simulink model "SensorTesting"  (R2025a)
settings: Solver=VariableStepAuto  StartTime=0.0  StopTime=10.0  RelTol=1e-3
undefined symbols (not defined in the file): fractalcoef
libraries: sensorgpslib x1, mspsensorlib x1, simulink x1
settings Model: Creator=jonno  LastModifiedBy=jonno

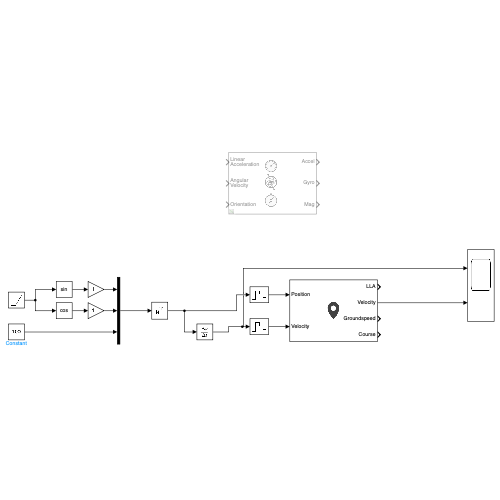
[thumbnail: Simulink's stored preview of the top-level diagram]
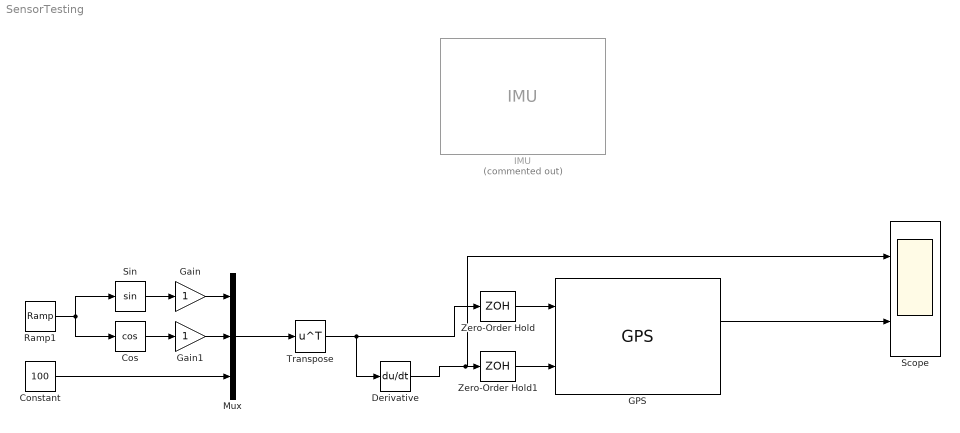
== system SensorTesting ==
  Constant : Constant  Value=100
  Cos : Trigonometry  Operator=cos
  Derivative : Derivative
  GPS : sensorgpslib/GPS  DispRefFrame=NED  PositionInputFormat=Local  ReferenceLocation=[ 0, 0, 0 ]  HorizontalPositionAccuracy=1.6  VerticalPositionAccuracy=3  VelocityAccuracy=0.1  DecayFactor=0.999  SeedDouble=67  SimulateUsing=Interpreted execution
      settings: LibrarySourceBlock=mspsensorlib/GPS
  Gain : Gain
  Gain1 : Gain
  IMU : mspsensorlib/IMU  Commented=on  DispRefFrame=NED  TemperaturePort=off  Temperature=25  MagneticFieldPort=off  MagneticFieldNED=[ 27.5550, -2.4169, -16.0849 ]  MagneticFieldENU=[ -2.4169, 27.5550, 16.0849 ]  SeedDouble=67  SimulateUsing=Interpreted execution  AccelParamsMeasurementRange=Inf  AccelParamsResolution=0  AccelParamsConstantBias=[ 0, 0, 0 ]  AccelParamsAxesMisalignment=[ 100, 0, 0; 0, 100, 0; 0, 0, 100 ]  AccelParamsNoiseDensity=[ 0, 0, 0 ]  AccelParamsBiasInstability=[ 0, 0, 0 ]  AccelParamsBiasInstabilityNumerator=fractalcoef().Numerator  AccelParamsBiasInstabilityDenominator=fractalcoef().Denominator  AccelParamsRandomWalk=[ 0, 0, 0 ]  AccelParamsNoiseType=double-sided  AccelParamsTemperatureBias=[ 0, 0, 0 ]  AccelParamsTemperatureScaleFactor=[ 0, 0, 0 ]  GyroParamsMeasurementRange=Inf  GyroParamsResolution=0  GyroParamsConstantBias=[ 0, 0, 0 ]  GyroParamsAxesMisalignment=[ 100, 0, 0; 0, 100, 0; 0, 0, 100 ]  GyroParamsAccelerationBias=[ 0, 0, 0 ]  GyroParamsNoiseDensity=[ 0, 0, 0 ]  GyroParamsBiasInstability=[ 0, 0, 0 ]  GyroParamsBiasInstabilityNumerator=fractalcoef().Numerator  GyroParamsBiasInstabilityDenominator=fractalcoef().Denominator  GyroParamsRandomWalk=[ 0, 0, 0 ]  GyroParamsNoiseType=double-sided  GyroParamsTemperatureBias=[ 0, 0, 0 ]  GyroParamsTemperatureScaleFactor=[ 0, 0, 0 ]  MagParamsMeasurementRange=Inf  MagParamsResolution=0  MagParamsConstantBias=[ 0, 0, 0 ]  MagParamsAxesMisalignment=[ 100, 0, 0; 0, 100, 0; 0, 0, 100 ]  MagParamsNoiseDensity=[ 0, 0, 0 ]  MagParamsBiasInstability=[ 0, 0, 0 ]  MagParamsBiasInstabilityNumerator=fractalcoef().Numerator  MagParamsBiasInstabilityDenominator=fractalcoef().Denominator  MagParamsRandomWalk=[ 0, 0, 0 ]  MagParamsNoiseType=double-sided  MagParamsTemperatureBias=[ 0, 0, 0 ]  MagParamsTemperatureScaleFactor=[ 0, 0, 0 ]
  Mux : Mux  Inputs=3
  Ramp1 : simulink/Sources/Ramp  slope=2  start=0  InitialOutput=0
  Scope : Scope  NumInputPorts=2
      settings: ActiveDisplayYMinimum=-2.4961806534301521  ActiveDisplayYMaximum=2.4995756281589059
  Sin : Trigonometry
  Transpose : Math  Operator=transpose
  Zero-Order Hold : ZeroOrderHold  SampleTime=0.1
  Zero-Order Hold1 : ZeroOrderHold  SampleTime=0.1
  wires:
  Sin/1 -> Gain/1
  Gain1/1 -> Mux/2
  Cos/1 -> Gain1/1
  Gain/1 -> Mux/1
  Ramp1/1 -> Cos/1, Sin/1
  Constant/1 -> Mux/3
  Derivative/1 -> Scope/1, Zero-Order Hold1/1
  Transpose/1 -> Zero-Order Hold/1, Derivative/1
  Mux/1 -> Transpose/1
  Zero-Order Hold/1 -> GPS/1
  Zero-Order Hold1/1 -> GPS/2
  GPS/2 -> Scope/2
